simulink model "NewHumanHandModel"  (R2013b)
settings: Solver=ode3  StartTime=0.0  StopTime=10.0  FixedStep=0.001  RelTol=1e-3
StopFcn:
  | position = posProfile.signals.values;
  | velocity = velProfile.signals.values;
  | diffPosition = diff(position);
  | diffPosition(diffPosition == 0) = [];
  | 
  | 
  | position(length(diffPosition): end)= []; %remove trailing zeros. neede for midi sound.
  | velocity(length(diffPosition): end) = [];
  | 
  | position = position'; velocity = velocity';
  | position(position ~= -0.2623) = 0;
  | position(position ~= 0) = 1;
  | 
  | num = 1:length(position);
  | posVel = [num; position; velocity];
  | fid = fopen('posVel.txt','w');
  | fprintf(fid, '%5d, %6.4f %6.4f;\n', posVel);
  | fclose(fid);
  | 
  | velocityMax = velocity(min(find(position == 1)));
  | velocityMin = velocity(max(find(position == 1)));
  | 
  | fid = fopen('minMax.txt', 'w');
  | fprintf(fid, '%1d, %6.4f %6.4f;\n', 1, velocityMin, velocityMax);
  | fclose(fid);
undefined symbols (not defined in the file): sigbuilder_block
settings Model: Creator=Deepak  LastModifiedBy=Deepak

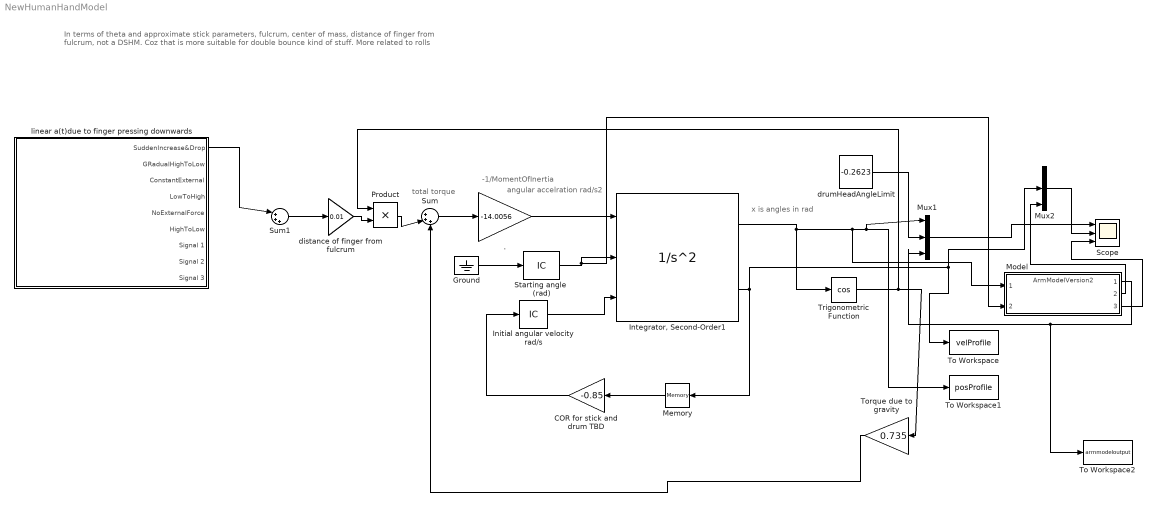
== system NewHumanHandModel ==
  note: total torque
  note: -1/MomentOfInertia
  note: x is angles in rad
  note: angular accelration rad/s2
  note: In terms of theta and approximate stick parameters, fulcrum, center of mass, distance of finger from fulcrum, not a DSHM. Coz that is more suitable for double bounce kind of stuff. More related to rolls
  . : Gain  Gain=-14.0056
  COR for stick and drum TBD : Gain  Gain=-0.85
  Ground : Ground
  "Initial angular velocity rad/s " : InitialCondition  Value=0
  "Integrator, Second-Order1" : SecondOrderIntegrator  ICSourceX=external  LimitX=on  LowerLimitX=-0.2623  ICSourceDXDT=external  ReinitDXDTwhenXreachesSaturation=on
  Memory : Memory
  Model : ModelReference  ModelNameDialog=ArmModelVersion2.slx  SimulationMode=Normal  ModelReferenceVersion=1.91  CopyOfModelName=ArmModelVersion2.slx  DefaultDataLogging=on
  Mux1 : Mux  Inputs=3
  Mux2 : Mux  Inputs=3
  Product : Product
  Scope : Scope  NumInputPorts=3
      settings: TimeRange=10  YMin=-1.8~-5~-5  YMax=0~5~5  MaxDataPoints=50000
  Starting angle  (rad) : InitialCondition  Value=0
  Sum : Sum  Inputs=|+++
  Sum1 : Sum  Inputs=|+++
  To Workspace : ToWorkspace  VariableName=velProfile  SampleTime=-1  SaveFormat=Structure
  To Workspace1 : ToWorkspace  VariableName=posProfile  SampleTime=-1  SaveFormat=Structure
  To Workspace2 : ToWorkspace  VariableName=armmodeloutput  SampleTime=-1  SaveFormat=Structure
  Torque due to gravity : Gain  Gain=0.735
  Trigonometric Function : Trigonometry  Operator=cos
  distance of finger from fulcrum : Gain  Gain=0.01
  drumHeadAngleLimit : Constant  Value=-0.2623
  linear a(t)due to finger pressing downwards : Subsystem  Tag=STV Subsys  LoadFcn=sigbuilder_block('load');  StartFcn=sigbuilder_block('start');  StopFcn=sigbuilder_block('stop');  ClipboardFcn=sigbuilder_block('clipboard');  mask(Sigbuilder block){}
      mask help: Simulink:masks:SigbuilderBlock_MD
      mask init:
      | if ~strcmp(get_param(bdroot(gcbh),'SimulationStatus'),'stopped') tuvar = sigbuilder_block('maskInit'); end
      settings: CopyFcn=sigbuilder_block('copy');  DeleteFcn=sigbuilder_block('delete');  ModelCloseFcn=sigbuilder_block('modelClose');  PreSaveFcn=sigbuilder_block('preSave');  PauseFcn=sigbuilder_block('pause');  ContinueFcn=sigbuilder_block('continue');  NameChangeFcn=sigbuilder_block('namechange');  OpenFcn=sigbuilder_block('open',[1259.01 352.722 549.567 545.57 ]);  CloseFcn=sigbuilder_block('close');
      mask Display: plot(0, 0, 100, 100,[2, 2, 32, 32, 2], [68, 8, 8, 68, 68],[32, 2], [38, 38], [32, 19, 2],[53, 60, 44], [32, 17, 17, 2],[16, 16, 31, 31]);txt = getActiveGroup(gcbh);text(2, 100, txt,'verticalAlignment', 'top');
  wires:
  "Integrator, Second-Order1"/1 -> Model/1, To Workspace1/1, Mux1/1, Trigonometric Function/1
  Trigonometric Function/1 -> Product/1, Torque due to gravity/1
  Sum/1 -> ./1
  Torque due to gravity/1 -> Sum/3
  Ground/1 -> Starting angle  (rad)/1
  Starting angle  (rad)/1 -> Model/2, "Integrator, Second-Order1"/2
  "Initial angular velocity rad/s "/1 -> "Integrator, Second-Order1"/3
  "Integrator, Second-Order1"/2 -> Memory/1, To Workspace/1, Mux2/2
  Memory/1 -> COR for stick and drum TBD/1
  COR for stick and drum TBD/1 -> "Initial angular velocity rad/s "/1
  Mux1/1 -> Scope/1
  drumHeadAngleLimit/1 -> Mux1/2
  distance of finger from fulcrum/1 -> Product/2
  Sum1/1 -> distance of finger from fulcrum/1
  Model/1 -> To Workspace2/1, Mux1/3
  Mux2/1 -> Scope/2
  Model/2 -> Mux2/3
  Model/3 -> Scope/3
  Product/1 -> Sum/2
  ./1 -> "Integrator, Second-Order1"/1
  linear a(t)due to finger pressing downwards/1(SuddenIncrease&Drop) -> Sum1/1

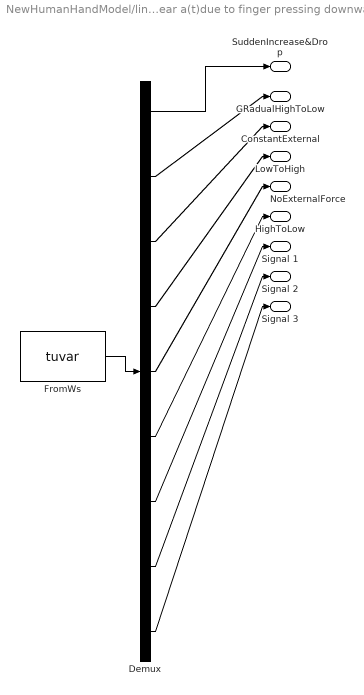
== system NewHumanHandModel/linear a(t)due to finger pressing downwards ==
  Demux : Demux  Tag=STV Demux  Outputs=9
  FromWs : FromWorkspace  Tag=STV FromWs  VariableName=tuvar  SampleTime=0
      SigBuilderData=|
      | common.afterFinalStr = 'Extrapolate'
      | common.sampleTime = 0
      | dataSet.timeRange = [0 10]
      | dataSet.name = 'Group 1'
      | sbobj.Groups.Name = 'Group 1'
      | sbobj.Groups.Signals(1).Name = 'SuddenIncrease&Drop'
      | sbobj.Groups.Signals(1).XData = [0 0.5 0.8 10]
      | sbobj.Groups.Signals(1).YData = [1 200 10 1]
      | sbobj.Groups.Signals(2).Name = 'GRadualHighToLow'
      | sbobj.Groups.Signals(2).XData = [0 10]
      | sbobj.Groups.Signals(2).YData = [100 1]
      | sbobj.Groups.Signals(3).Name = 'ConstantExternal'
      | sbobj.Groups.Signals(3).XData = [0 10]
      | sbobj.Groups.Signals(3).YData = [89.05 89.05]
      | sbobj.Groups.Signals(4).Name = 'LowToHigh'
      | sbobj.Groups.Signals(4).XData = [0 1.1 1.5 10]
      | sbobj.Groups.Signals(4).YData = [1 1 200 10]
      | sbobj.Groups.Signals(5).Name = 'NoExternalForce'
      | sbobj.Groups.Signals(5).XData = [0 10]
      | sbobj.Groups.Signals(5).YData = [0 0]
      | sbobj.Groups.Signals(6).Name = 'HighToLow'
      | sbobj.Groups.Signals(6).XData = [0 0.5 0.6 0.6 10]
      | sbobj.Groups.Signals(6).YData = [200 200 5 0 -10]
      | sbobj.Groups.Signals(7).Name = 'Signal 1'
      | sbobj.Groups.Signals(7).XData = [0 0.6 0.6 0.62 0.62 10]
      | sbobj.Groups.Signals(7).YData = [0 0 200 200 0 0]
      | sbobj.Groups.Signals(8).Name = 'Signal 2'
      | sbobj.Groups.Signals(8).XData = [0 1.18 1.18 1.22 1.22 10]
      | sbobj.Groups.Signals(8).YData = [0 0 300 300 0 0]
      | sbobj.Groups.Signals(9).Name = 'Signal 3'
      | sbobj.Groups.Signals(9).XData = [0 10]
      | sbobj.Groups.Signals(9).YData = [-73.5 -73.5]
  SuddenIncrease&Drop : Outport  Tag=STV Outport
  GRadualHighToLow : Outport  Tag=STV Outport  Port=2
  ConstantExternal : Outport  Tag=STV Outport  Port=3
  LowToHigh : Outport  Tag=STV Outport  Port=4
  NoExternalForce : Outport  Tag=STV Outport  Port=5
  HighToLow : Outport  Tag=STV Outport  Port=6
  Signal 1 : Outport  Tag=STV Outport  Port=7
  Signal 2 : Outport  Tag=STV Outport  Port=8
  Signal 3 : Outport  Tag=STV Outport  Port=9
  wires:
  Demux/3 -> ConstantExternal/1
  Demux/2 -> GRadualHighToLow/1
  Demux/1 -> SuddenIncrease&Drop/1
  FromWs/1 -> Demux/1
  Demux/4 -> LowToHigh/1
  Demux/5 -> NoExternalForce/1
  Demux/6 -> HighToLow/1
  Demux/7 -> Signal 1/1
  Demux/8 -> Signal 2/1
  Demux/9 -> Signal 3/1
